simulink model "BrakingDyn"  (R2014b)
settings: Solver=ode45  StartTime=0.0  StopTime=10.0  RelTol=1e-3
undefined symbols (not defined in the file): a, Area_BrakePad, BrakeDiscRaduis, C_a, FrictionCoefficient_BrakeDisc, g, h, k_brake_pressure, l, l_f, p_max, p_min, r_wheel, rho
settings Model: RequirementInfo="{}  %GIDa_9f951571_3c7b_457f_a1ff_dbbb27cc037c"  Creator=putta  LastModifiedBy=putta

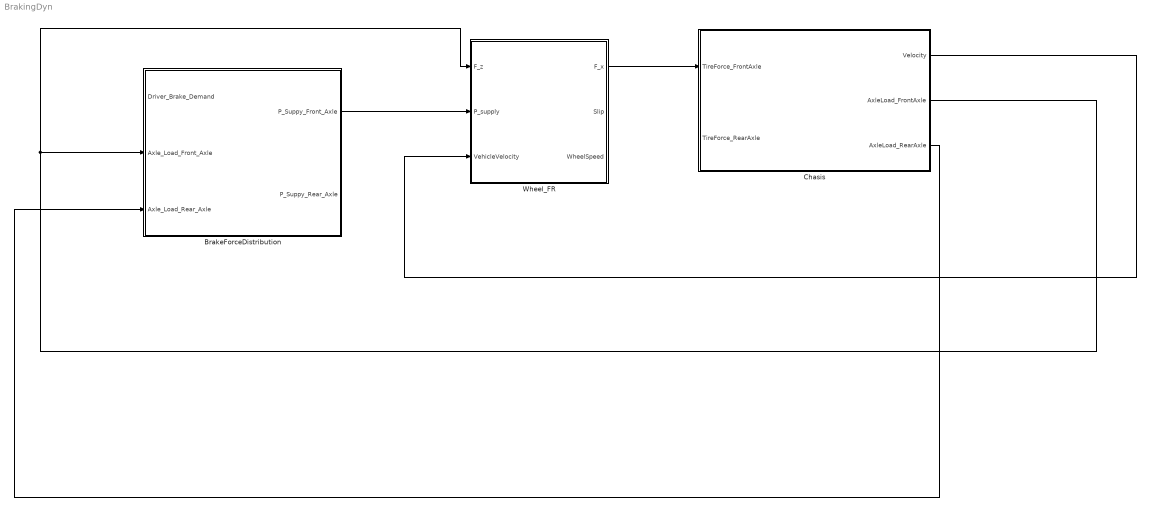
== system BrakingDyn ==
  BrakeForceDistribution : Subsystem
  Chasis : Subsystem
  Wheel_FR : Subsystem
  wires:
  Chasis/1(Velocity) -> Wheel_FR/3(VehicleVelocity)
  Wheel_FR/1(F_x) -> Chasis/1(TireForce_FrontAxle)
  BrakeForceDistribution/1(P_Suppy_Front_Axle) -> Wheel_FR/2(P_supply)
  Chasis/2(AxleLoad_FrontAxle) -> Wheel_FR/1(F_z), BrakeForceDistribution/2(Axle_Load_Front_Axle)
  Chasis/3(AxleLoad_RearAxle) -> BrakeForceDistribution/3(Axle_Load_Rear_Axle)

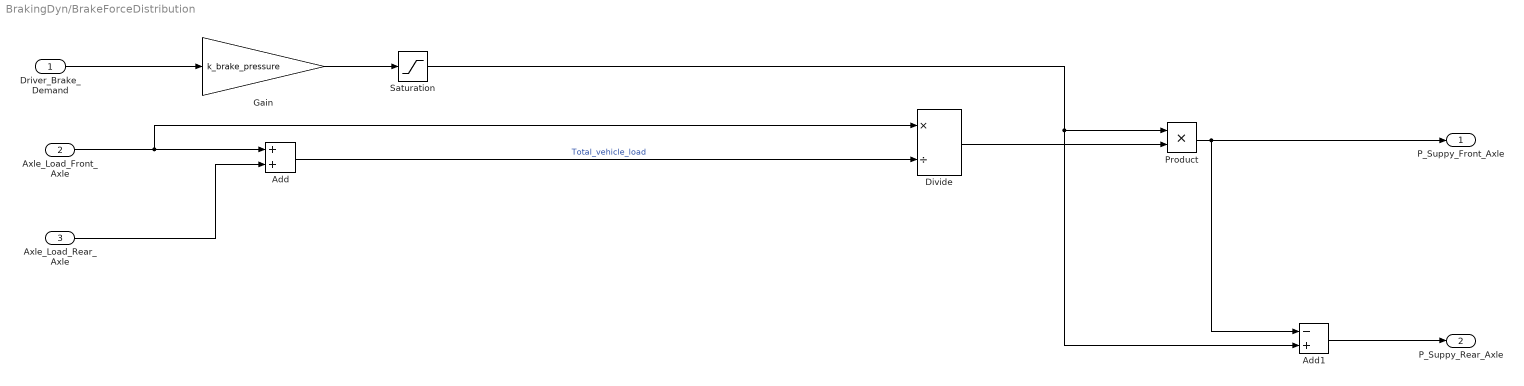
== system BrakingDyn/BrakeForceDistribution ==
  Driver_Brake_Demand : Inport
  Axle_Load_Front_Axle : Inport  Port=2
  Axle_Load_Rear_Axle : Inport  Port=3
  Add : Sum
  Add1 : Sum  Inputs=-+
  Divide : Product  Inputs=*/
  Gain : Gain  Gain=k_brake_pressure
  Product : Product
  Saturation : Saturate  UpperLimit=p_max  LowerLimit=p_min
  P_Suppy_Front_Axle : Outport
  P_Suppy_Rear_Axle : Outport  Port=2
  wires:
  Driver_Brake_Demand/1 -> Gain/1
  Gain/1 -> Saturation/1
  Axle_Load_Front_Axle/1 -> Divide/1, Add/1
  Axle_Load_Rear_Axle/1 -> Add/2
  Add/1 -> Divide/2  "Total_vehicle_load"
  Divide/1 -> Product/2
  Saturation/1 -> Add1/2, Product/1
  Product/1 -> Add1/1, P_Suppy_Front_Axle/1
  Add1/1 -> P_Suppy_Rear_Axle/1

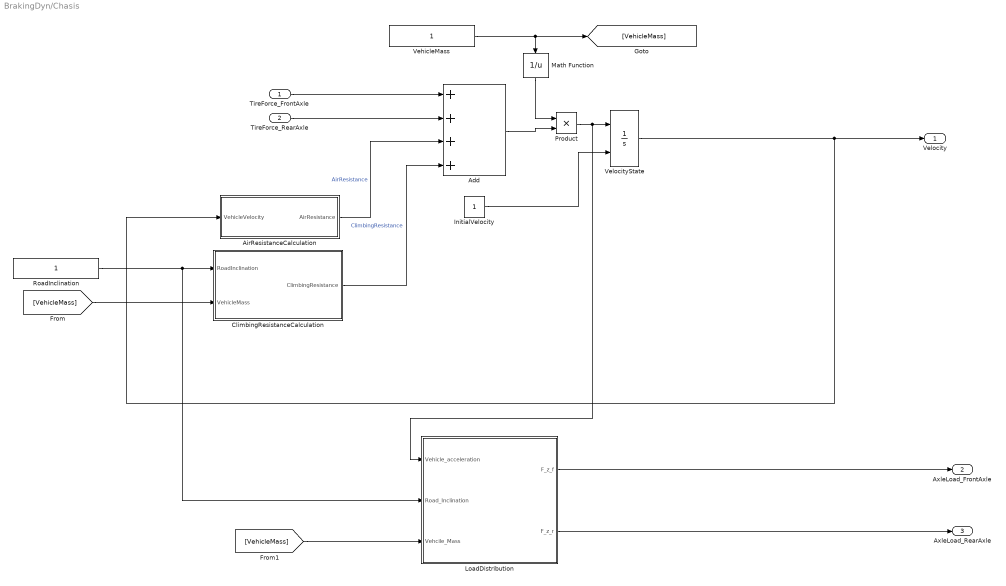
== system BrakingDyn/Chasis ==
  TireForce_FrontAxle : Inport
  TireForce_RearAxle : Inport  Port=2
  Add : Sum  Inputs=++++
  AirResistanceCalculation : Subsystem
  ClimbingResistanceCalculation : Subsystem
  "InitialVelocity " : Constant
  LoadDistribution : Subsystem
  Math Function : Math  Operator=reciprocal  SaturateOnIntegerOverflow=on
  Product : Product
  RoadInclination : Constant
  "VehicleMass " : Constant
  VelocityState : Integrator  InitialConditionSource=external
  Velocity : Outport
  AxleLoad_FrontAxle : Outport  Port=2
  AxleLoad_RearAxle : Outport  Port=3
  wires:
  "InitialVelocity "/1 -> VelocityState/2
  TireForce_FrontAxle/1 -> Add/1
  TireForce_RearAxle/1 -> Add/2
  AirResistanceCalculation/1(AirResistance) -> Add/3  "AirResistance"
  ClimbingResistanceCalculation/1(ClimbingResistance) -> Add/4  "ClimbingResistance"
  VelocityState/1 -> AirResistanceCalculation/1(VehicleVelocity), Velocity/1
  Product/1 -> LoadDistribution/1(Vehicle_acceleration), VelocityState/1
  Add/1 -> Product/2
  "VehicleMass "/1 -> Math Function/1, [VehicleMass]
  RoadInclination/1 -> LoadDistribution/2(Road_Inclination), ClimbingResistanceCalculation/1(RoadInclination)
  [VehicleMass] -> ClimbingResistanceCalculation/2(VehicleMass)
  LoadDistribution/1(F_z_f) -> AxleLoad_FrontAxle/1
  LoadDistribution/2(F_z_r) -> AxleLoad_RearAxle/1
  Math Function/1 -> Product/1
  [VehicleMass] -> LoadDistribution/3(Vehcile_Mass)

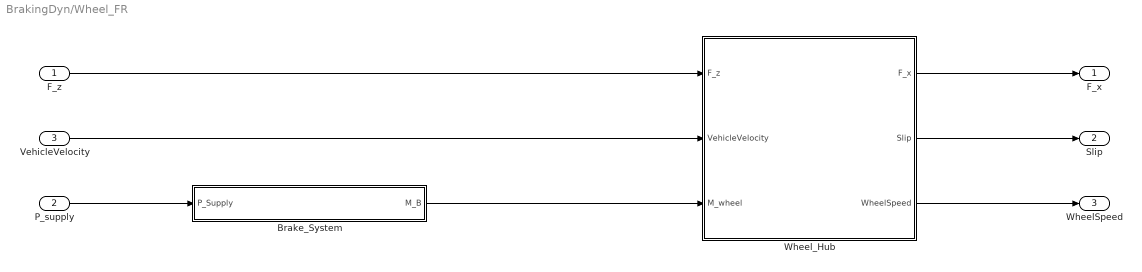
== system BrakingDyn/Wheel_FR ==
  F_z : Inport
  P_supply : Inport  Port=2
  VehicleVelocity : Inport  Port=3
  Brake_System : Subsystem
  Wheel_Hub : Subsystem
  F_x : Outport
  Slip : Outport  Port=2
  WheelSpeed : Outport  Port=3
  wires:
  F_z/1 -> Wheel_Hub/1(F_z)
  VehicleVelocity/1 -> Wheel_Hub/2(VehicleVelocity)
  Wheel_Hub/1(F_x) -> F_x/1
  Wheel_Hub/2(Slip) -> Slip/1
  Wheel_Hub/3(WheelSpeed) -> WheelSpeed/1
  P_supply/1 -> Brake_System/1(P_Supply)
  Brake_System/1(M_B) -> Wheel_Hub/3(M_wheel)

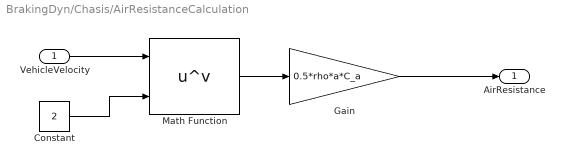
== system BrakingDyn/Chasis/AirResistanceCalculation ==
  VehicleVelocity : Inport
  Constant : Constant  Value=2
  Gain : Gain  Gain=0.5*rho*a*C_a
  Math Function : Math  Operator=pow  SaturateOnIntegerOverflow=on
  AirResistance : Outport
  wires:
  Gain/1 -> AirResistance/1
  Math Function/1 -> Gain/1
  VehicleVelocity/1 -> Math Function/1
  Constant/1 -> Math Function/2

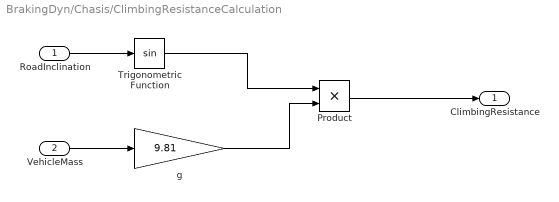
== system BrakingDyn/Chasis/ClimbingResistanceCalculation ==
  RoadInclination : Inport
  VehicleMass : Inport  Port=2
  Product : Product
  Trigonometric Function : Trigonometry
  g : Gain  Gain=9.81
  ClimbingResistance : Outport
  wires:
  VehicleMass/1 -> g/1
  RoadInclination/1 -> Trigonometric Function/1
  Product/1 -> ClimbingResistance/1
  Trigonometric Function/1 -> Product/1
  g/1 -> Product/2

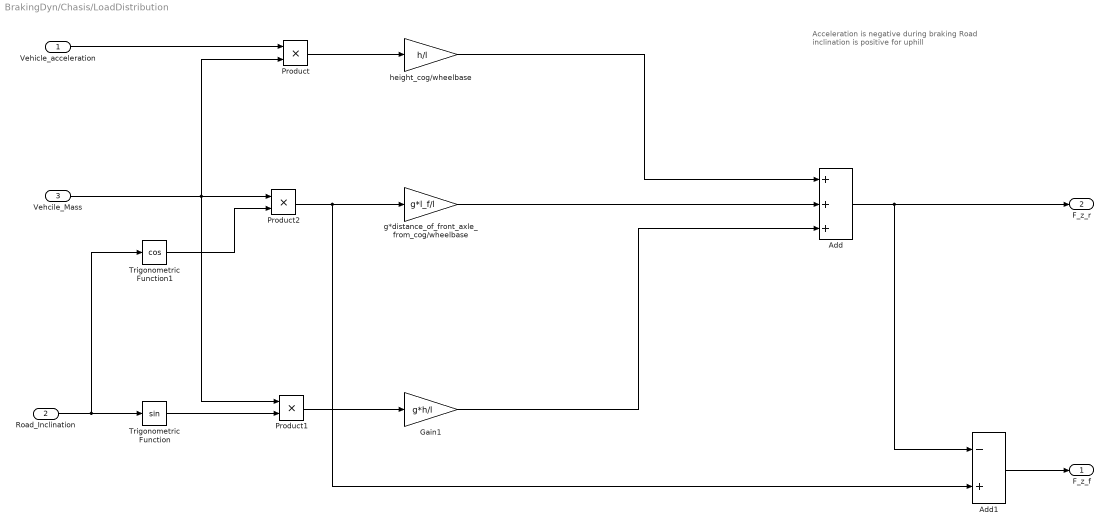
== system BrakingDyn/Chasis/LoadDistribution ==
  note: Acceleration is negative during braking
      | Road inclination is positive for uphill
  Vehicle_acceleration : Inport
  Road_Inclination : Inport  Port=2
  Vehcile_Mass : Inport  Port=3
  Add : Sum  Inputs=+++
  Add1 : Sum  Inputs=-+
  Gain1 : Gain  Gain=g*h/l
  Product : Product
  Product1 : Product
  Product2 : Product
  Trigonometric Function : Trigonometry
  Trigonometric Function1 : Trigonometry  Operator=cos
  g*distance_of_front_axle_from_cog/wheelbase : Gain  Gain=g*l_f/l
  height_cog/wheelbase : Gain  Gain=h/l
  F_z_f : Outport
  F_z_r : Outport  Port=2
  wires:
  Vehcile_Mass/1 -> Product/2, Product2/1, Product1/1
  Product/1 -> height_cog/wheelbase/1
  Vehicle_acceleration/1 -> Product/1
  Road_Inclination/1 -> Trigonometric Function1/1, Trigonometric Function/1
  Product1/1 -> Gain1/1
  Trigonometric Function/1 -> Product1/2
  Product2/1 -> Add1/2, g*distance_of_front_axle_from_cog/wheelbase/1
  Trigonometric Function1/1 -> Product2/2
  height_cog/wheelbase/1 -> Add/1
  g*distance_of_front_axle_from_cog/wheelbase/1 -> Add/2
  Gain1/1 -> Add/3
  Add/1 -> Add1/1, F_z_r/1
  Add1/1 -> F_z_f/1

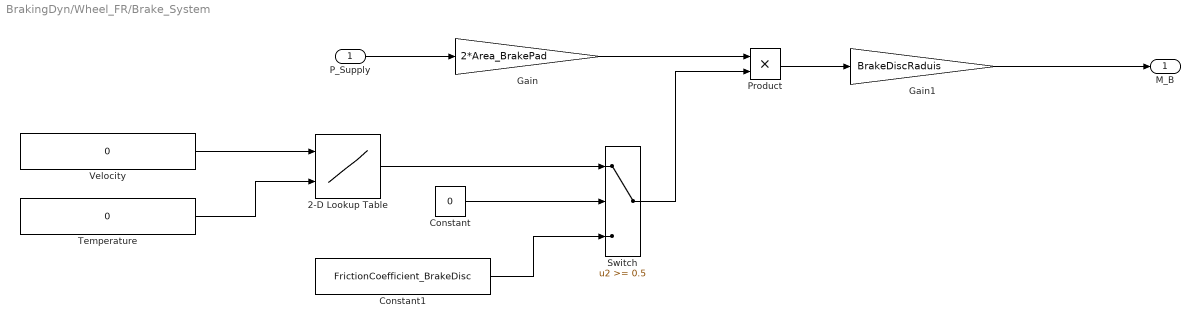
== system BrakingDyn/Wheel_FR/Brake_System ==
  P_Supply : Inport
  2-D Lookup Table : Lookup_n-D  BreakpointsForDimension1=[1:3]  BreakpointsForDimension2=[1:3]  InternalRulePriority=Speed  RndMeth=Simplest  InputSameDT=on
  Constant : Constant  Value=0
  Constant1 : Constant  Value=FrictionCoefficient_BrakeDisc
  Gain : Gain  Gain=2*Area_BrakePad
  Gain1 : Gain  Gain=BrakeDiscRaduis
  Product : Product
  Switch : Switch  Threshold=0.5
      settings: AttributesFormatString=criteria=%<Criteria>\nthreshold=%<Threshold>
  Temperature : Constant  Value=0
  Velocity : Constant  Value=0
  M_B : Outport
  wires:
  P_Supply/1 -> Gain/1
  Gain/1 -> Product/1
  Switch/1 -> Product/2
  Constant1/1 -> Switch/3
  Constant/1 -> Switch/2
  2-D Lookup Table/1 -> Switch/1
  Velocity/1 -> 2-D Lookup Table/1
  Temperature/1 -> 2-D Lookup Table/2
  Product/1 -> Gain1/1
  Gain1/1 -> M_B/1

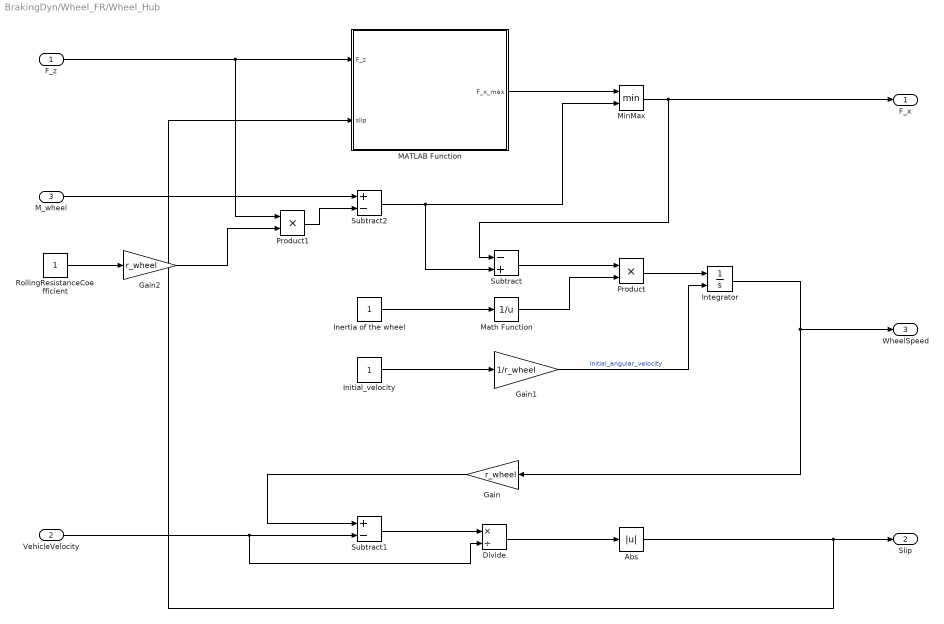
== system BrakingDyn/Wheel_FR/Wheel_Hub ==
  F_z : Inport
  VehicleVelocity : Inport  Port=2
  M_wheel : Inport  Port=3
  Abs : Abs
  Divide : Product  Inputs=*/
  Gain : Gain  Gain=r_wheel
  Gain1 : Gain  Gain=1/r_wheel
  Gain2 : Gain  Gain=r_wheel
  Inertia of the wheel : Constant
  Initial_velocity : Constant
  Integrator : Integrator  InitialConditionSource=external
  MATLAB Function : MATLAB Function  TreatAsAtomicUnit=on
  Math Function : Math  Operator=reciprocal  SaturateOnIntegerOverflow=on
  MinMax : MinMax  Inputs=2
  Product : Product
  Product1 : Product
  RollingResistanceCoefficient : Constant
  Subtract : Sum  Inputs=-+
  Subtract1 : Sum  Inputs=+-
  Subtract2 : Sum  Inputs=+-
  F_x : Outport
  Slip : Outport  Port=2
  WheelSpeed : Outport  Port=3
  wires:
  MATLAB Function/1(F_x_max) -> MinMax/1
  Subtract/1 -> Product/1
  Math Function/1 -> Product/2
  MinMax/1 -> F_x/1, Subtract/1
  F_z/1 -> Product1/1, MATLAB Function/1(F_z)
  VehicleVelocity/1 -> Subtract1/2, Divide/2
  Divide/1 -> Abs/1
  Initial_velocity/1 -> Gain1/1
  M_wheel/1 -> Subtract2/1
  Product1/1 -> Subtract2/2
  Gain/1 -> Subtract1/1
  Product/1 -> Integrator/1
  Gain1/1 -> Integrator/2  "Initial_angular_velocity"
  Subtract2/1 -> Subtract/2, MinMax/2
  Integrator/1 -> WheelSpeed/1, Gain/1
  RollingResistanceCoefficient/1 -> Gain2/1
  Subtract1/1 -> Divide/1
  Inertia of the wheel/1 -> Math Function/1
  Abs/1 -> Slip/1, MATLAB Function/2(slip)
  Gain2/1 -> Product1/2

== matlab function BrakingDyn/Wheel_FR/Wheel_Hub/MATLAB Function ==
  data: F_z input; slip input; F_x_max output
function F_x_max = fcn(F_z,slip)
%#codegen
s = slip;
F_x_max = F_z*D*sin(C*atan((B*s-E*(B*s-atan(B*s)))));
